simulink model "Switch"  (R2024b)
settings: Solver=VariableStepAuto  StartTime=0.0  StopTime=10.0  RelTol=1e-3
settings Model: Creator=abdal  LastModifiedBy=abdal

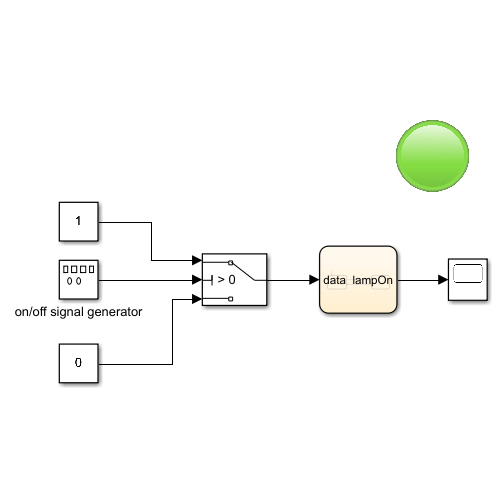
[thumbnail: Simulink's stored preview of the top-level diagram]
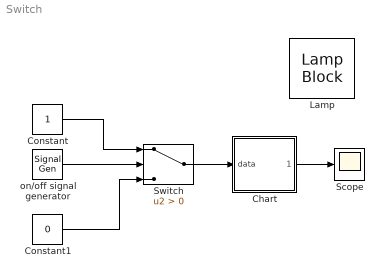
== system Switch ==
  Chart : Stateflow chart  TreatAsAtomicUnit=on
  Constant : Constant
  Constant1 : Constant  Value=0
  Lamp : LampBlock  LabelPosition=Hide
  Scope : Scope
  Switch : Switch  Criteria=u2 > Threshold  SaturateOnIntegerOverflow=off  InputSameDT=off
  on/off signal generator : SignalGenerator  Units=rad/sec
  wires:
  Constant/1 -> Switch/1
  on/off signal generator/1 -> Switch/2
  Switch/1 -> Chart/1(data)
  Constant1/1 -> Switch/3
  Chart/1(lampOn) -> Scope/1

== stateflow chart Switch/Chart ==
  state On
    entry:
    lampOn = 1;
  state Off
    entry:
    lampOn = 0;
  (default) -> On
  On -> Off : [data == 0]
  Off -> On : [data == 1]
  data: data input; lampOn output
